simulink model "Three_phase_transformer_simulation"  (R2013b)
settings: Solver=ode45  StartTime=0.0  StopTime=0.1  RelTol=1e-3
libraries: powerlib x123
settings Model: Creator=Talha Israr  LastModifiedBy=Talha Israr

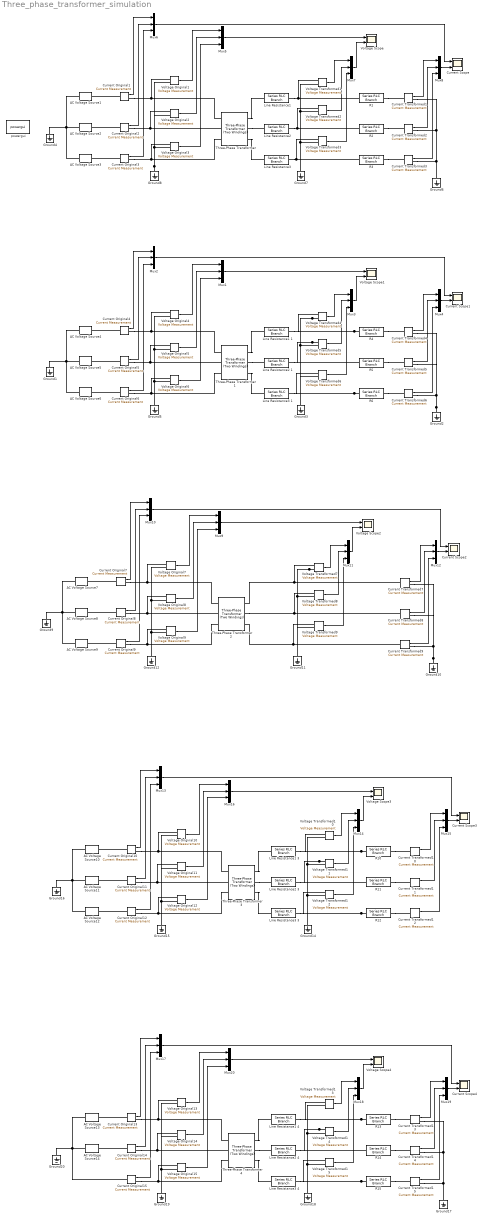
== system Three_phase_transformer_simulation ==
  AC Voltage Source{1,4,7,10,13} (5 alike) : powerlib/Electrical Sources/AC Voltage Source  Amplitude=220  Phase=0  Frequency=50  SampleTime=0  Measurements=None
  AC Voltage Source{2,5,8,11,14} (5 alike) : powerlib/Electrical Sources/AC Voltage Source  Amplitude=220  Phase=120  Frequency=50  SampleTime=0  Measurements=None
  AC Voltage Source{3,6,9,12} (4 alike) : powerlib/Electrical Sources/AC Voltage Source  Amplitude=220  Phase=240  Frequency=50  SampleTime=0  Measurements=None
  Current Original{1..15} (15 alike) : powerlib/Measurements/Current Measurement  PhasorSimulation=off  OutputType=Complex  PSBequivalent=0
  Current Scope{,1..4} (5 alike) : Scope  NumInputPorts=2
      Current Scope settings: YMin=-225~-1.25  YMax=300~1.5  MaxDataPoints=300000
      Current Scope1 settings: YMin=-225~-1.25  YMax=300~1.5  SaveName=ScopeData2  MaxDataPoints=300000
      Current Scope2 settings: YMin=-225~-1.25  YMax=300~1.5  SaveName=ScopeData4  MaxDataPoints=300000
      Current Scope3 settings: YMin=-225~-1.25  YMax=300~1.5  SaveName=ScopeData6  MaxDataPoints=300000
      Current Scope4 settings: YMin=-225~-1.25  YMax=300~1.5  SaveName=ScopeData8  MaxDataPoints=300000
  Current Transformed{1..15} (15 alike) : powerlib/Measurements/Current Measurement  PhasorSimulation=off  OutputType=Complex  PSBequivalent=0
  Ground{1..12,14..20} (19 alike) : powerlib/Elements/Ground  LConnTagsString=a
  Line Resistance1 {,1,3..4} (4 alike) : powerlib/Elements/Series RLC Branch  LConnTagsString=__new0  RConnTagsString=__new0  BranchType=R  Resistance=5  Inductance=1e-3  SetiL0=off  InitialCurrent=0  Capacitance=1e-6  Setx0=off  InitialVoltage=0  Measurements=None
  Line Resistance2 {,1,3..4} (4 alike) : powerlib/Elements/Series RLC Branch  LConnTagsString=__new0  RConnTagsString=__new0  BranchType=R  Resistance=5  Inductance=1e-3  SetiL0=off  InitialCurrent=0  Capacitance=1e-6  Setx0=off  InitialVoltage=0  Measurements=None
  Line Resistance3 {,1,3..4} (4 alike) : powerlib/Elements/Series RLC Branch  LConnTagsString=__new0  RConnTagsString=__new0  BranchType=R  Resistance=5  Inductance=2e-3  SetiL0=off  InitialCurrent=0  Capacitance=1e-6  Setx0=off  InitialVoltage=0  Measurements=None
  Mux{1..20} (20 alike) : Mux  Inputs=3
  R{1..2,10..11,13..14} (6 alike) : powerlib/Elements/Series RLC Branch  LConnTagsString=__new0  RConnTagsString=__new0  BranchType=R  Resistance=100  Inductance=1e-3  SetiL0=off  InitialCurrent=0  Capacitance=1e-6  Setx0=off  InitialVoltage=0  Measurements=None
  R12 : powerlib/Elements/Series RLC Branch  LConnTagsString=__new0  RConnTagsString=__new0  BranchType=R  Resistance=100  Inductance=2e-3  SetiL0=off  InitialCurrent=0  Capacitance=1e-6  Setx0=off  InitialVoltage=0  Measurements=None
  R15 : powerlib/Elements/Series RLC Branch  LConnTagsString=__new0  RConnTagsString=__new0  BranchType=R  Resistance=100  Inductance=2e-3  SetiL0=off  InitialCurrent=0  Capacitance=1e-6  Setx0=off  InitialVoltage=0  Measurements=None
  R3 : powerlib/Elements/Series RLC Branch  LConnTagsString=__new0  RConnTagsString=__new0  BranchType=R  Resistance=100  Inductance=2e-3  SetiL0=off  InitialCurrent=0  Capacitance=1e-6  Setx0=off  InitialVoltage=0  Measurements=None
  R4 : powerlib/Elements/Series RLC Branch  LConnTagsString=__new0  RConnTagsString=__new0  BranchType=RLC  Resistance=100  Inductance=5e-3  SetiL0=off  InitialCurrent=0  Capacitance=2e-6  Setx0=off  InitialVoltage=0  Measurements=None
  R5 : powerlib/Elements/Series RLC Branch  LConnTagsString=__new0  RConnTagsString=__new0  BranchType=RLC  Resistance=100  Inductance=5e-3  SetiL0=off  InitialCurrent=0  Capacitance=2e-6  Setx0=off  InitialVoltage=0  Measurements=None
  R6 : powerlib/Elements/Series RLC Branch  LConnTagsString=__new0  RConnTagsString=__new0  BranchType=RLC  Resistance=100  Inductance=5e-3  SetiL0=off  InitialCurrent=0  Capacitance=2e-6  Setx0=off  InitialVoltage=0  Measurements=None
  Three-Phase Transformer {,1..2,4} (4 alike) : powerlib/Elements/Three-Phase Transformer (Two Windings)  Winding1Connection=Y  UNITS=pu  NominalPower=[ 250e6 , 60 ]  Winding1=[ 220e3 , 0.002 , 0.08 ]  Winding2Connection=Y  Winding2=[ 12e3 , 0.002 , 0.08 ]  SetSaturation=off  Rm=500  Lm=500  Saturation=[ 0,0 ; 0.0024,1.2 ; 1.0,1.52 ]  Hysteresis=off  DataFile='hysteresis'  SetInitialFlux=off  InitialFluxes=[ 0.8 , -0.8 , 0.7 ]  Measurements=None  MoreParameters=off  BreakLoop=off  DataType=off  TransfoNumber=1
  Three-Phase Transformer 3 : powerlib/Elements/Three-Phase Transformer (Two Windings)  Winding1Connection=Yg  UNITS=pu  NominalPower=[ 250e6 , 60 ]  Winding1=[ 220e3 , 0.002 , 0.08 ]  Winding2Connection=Yg  Winding2=[ 12e3 , 0.002 , 0.08 ]  SetSaturation=off  Rm=500  Lm=500  Saturation=[ 0,0 ; 0.0024,1.2 ; 1.0,1.52 ]  Hysteresis=off  DataFile='hysteresis'  SetInitialFlux=off  InitialFluxes=[ 0.8 , -0.8 , 0.7 ]  Measurements=None  MoreParameters=off  BreakLoop=off  DataType=off  TransfoNumber=1
  Voltage Original{1..15} (15 alike) : powerlib/Measurements/Voltage Measurement  PhasorSimulation=off  OutputType=Complex  PSBequivalent=0
  Voltage Scope{,1..4} (5 alike) : Scope  NumInputPorts=2
      Voltage Scope settings: YMin=-225~-1.25  YMax=300~1.5  MaxDataPoints=300000
      Voltage Scope1 settings: YMin=-225~-1.25  YMax=300~1.5  SaveName=ScopeData3  MaxDataPoints=300000
      Voltage Scope2 settings: YMin=-225~-1.25  YMax=300~1.5  SaveName=ScopeData5  MaxDataPoints=300000
      Voltage Scope3 settings: YMin=-225~-1.25  YMax=300~1.5  SaveName=ScopeData7  MaxDataPoints=300000
      Voltage Scope4 settings: YMin=-225~-1.25  YMax=300~1.5  SaveName=ScopeData9  MaxDataPoints=300000
  Voltage Transformed{1..15} (15 alike) : powerlib/Measurements/Voltage Measurement  PhasorSimulation=off  OutputType=Complex  PSBequivalent=0
  powergui : powerlib/powergui  Priority=1  SimulationMode=Continuous  SolverType=Tustin  SampleTime=50e-6  frequency=60  SPID=off  DisableSnubberDevices=off  DisableRonSwitches=off  DisableVfSwitches=off  SwTol=0  Interpol=off  DisplayEquations=off  frequencyindice=50  Pbase=100e6  ErrMax=1e-4  Iterations=50  UnitsV=kV  UnitsW=MW  FunctionMessages=off  echomessages=off  HookPort=off  EnableUseOfTLC=off  x0status=blocks  RestoreLinks=warning  ResistiveCurrentMeasurement=off  Frange=[0:2:500]  Ylog=off  Xlog=on  ShowGrid=off  save=off  variable=ZData  ZoomFFT=off  StartTime=0.0  cycles=1  DisplayStyle=1  fundamental=60  FreqAxis=off  MaxFrequency=1000  frequencyindicesteady=1  RmsSteady=1  display=off  Ts=0  methode=off
  wires:
  Current Original1/1 -> Mux6/1
  Current Original2/1 -> Mux6/2
  Current Original3/1 -> Mux6/3
  Voltage Transformed1/1 -> Mux7/1
  Voltage Transformed2/1 -> Mux7/2
  Voltage Transformed3/1 -> Mux7/3
  Current Transformed3/1 -> Mux8/3
  Current Transformed2/1 -> Mux8/2
  Current Transformed1/1 -> Mux8/1
  Mux6/1 -> Current Scope/1
  Mux8/1 -> Current Scope/2
  Mux5/1 -> Voltage Scope/1
  Mux7/1 -> Voltage Scope/2
  Voltage Original3/1 -> Mux5/3
  Voltage Original2/1 -> Mux5/2
  Voltage Original1/1 -> Mux5/1
  Current Original4/1 -> Mux2/1
  Current Original5/1 -> Mux2/2
  Current Original6/1 -> Mux2/3
  Voltage Transformed4/1 -> Mux3/1
  Voltage Transformed5/1 -> Mux3/2
  Voltage Transformed6/1 -> Mux3/3
  Current Transformed6/1 -> Mux4/3
  Current Transformed5/1 -> Mux4/2
  Current Transformed4/1 -> Mux4/1
  Mux2/1 -> Current Scope1/1
  Mux4/1 -> Current Scope1/2
  Mux1/1 -> Voltage Scope1/1
  Mux3/1 -> Voltage Scope1/2
  Voltage Original6/1 -> Mux1/3
  Voltage Original5/1 -> Mux1/2
  Voltage Original4/1 -> Mux1/1
  Current Original7/1 -> Mux10/1
  Current Original8/1 -> Mux10/2
  Current Original9/1 -> Mux10/3
  Voltage Transformed7/1 -> Mux11/1
  Voltage Transformed8/1 -> Mux11/2
  Voltage Transformed9/1 -> Mux11/3
  Current Transformed9/1 -> Mux12/3
  Current Transformed8/1 -> Mux12/2
  Current Transformed7/1 -> Mux12/1
  Mux10/1 -> Current Scope2/1
  Mux12/1 -> Current Scope2/2
  Mux9/1 -> Voltage Scope2/1
  Mux11/1 -> Voltage Scope2/2
  Voltage Original9/1 -> Mux9/3
  Voltage Original8/1 -> Mux9/2
  Voltage Original7/1 -> Mux9/1
  Current Original10/1 -> Mux13/1
  Current Original11/1 -> Mux13/2
  Current Original12/1 -> Mux13/3
  Voltage Transformed10/1 -> Mux14/1
  Voltage Transformed11/1 -> Mux14/2
  Voltage Transformed12/1 -> Mux14/3
  Current Transformed12/1 -> Mux15/3
  Current Transformed11/1 -> Mux15/2
  Current Transformed10/1 -> Mux15/1
  Mux13/1 -> Current Scope3/1
  Mux15/1 -> Current Scope3/2
  Mux16/1 -> Voltage Scope3/1
  Mux14/1 -> Voltage Scope3/2
  Voltage Original12/1 -> Mux16/3
  Voltage Original11/1 -> Mux16/2
  Voltage Original10/1 -> Mux16/1
  Current Original13/1 -> Mux17/1
  Current Original14/1 -> Mux17/2
  Current Original15/1 -> Mux17/3
  Voltage Transformed13/1 -> Mux18/1
  Voltage Transformed14/1 -> Mux18/2
  Voltage Transformed15/1 -> Mux18/3
  Current Transformed15/1 -> Mux19/3
  Current Transformed14/1 -> Mux19/2
  Current Transformed13/1 -> Mux19/1
  Mux17/1 -> Current Scope4/1
  Mux19/1 -> Current Scope4/2
  Mux20/1 -> Voltage Scope4/1
  Mux18/1 -> Voltage Scope4/2
  Voltage Original15/1 -> Mux20/3
  Voltage Original14/1 -> Mux20/2
  Voltage Original13/1 -> Mux20/1
  connections:
  R2/LConn1 -- "Line Resistance2 "/RConn1 -- Voltage Transformed2/LConn1
  AC Voltage Source2/LConn1 -- Ground4/LConn1 -- AC Voltage Source3/LConn1 -- AC Voltage Source1/LConn1
  Current Transformed1/RConn1 -- Current Transformed2/RConn1 -- Current Transformed3/RConn1 -- Ground6/LConn1
  Voltage Transformed3/LConn2 -- Ground7/LConn1 -- Voltage Transformed2/LConn2 -- Voltage Transformed1/LConn2
  Voltage Original2/LConn1 -- "Three-Phase Transformer "/LConn2 -- Current Original2/RConn1
  "Three-Phase Transformer "/LConn3 -- Voltage Original3/LConn1 -- Current Original3/RConn1
  Voltage Original1/LConn1 -- "Three-Phase Transformer "/LConn1 -- Current Original1/RConn1
  Voltage Transformed1/LConn1 -- "Line Resistance1 "/RConn1 -- R1/LConn1
  Ground8/LConn1 -- Voltage Original3/LConn2 -- Voltage Original1/LConn2 -- Voltage Original2/LConn2
  Current Original1/LConn1 -- AC Voltage Source1/RConn1
  R3/RConn1 -- Current Transformed3/LConn1
  R2/RConn1 -- Current Transformed2/LConn1
  Current Original2/LConn1 -- AC Voltage Source2/RConn1
  Voltage Transformed3/LConn1 -- "Line Resistance3 "/RConn1 -- R3/LConn1
  Current Original3/LConn1 -- AC Voltage Source3/RConn1
  R1/RConn1 -- Current Transformed1/LConn1
  "Three-Phase Transformer "/RConn2 -- "Line Resistance2 "/LConn1
  "Three-Phase Transformer "/RConn3 -- "Line Resistance3 "/LConn1
  "Three-Phase Transformer "/RConn1 -- "Line Resistance1 "/LConn1
  Voltage Transformed5/LConn1 -- R5/LConn1 -- Line Resistance2 1/RConn1
  AC Voltage Source4/LConn1 -- AC Voltage Source5/LConn1 -- Ground1/LConn1 -- AC Voltage Source6/LConn1
  Ground2/LConn1 -- Current Transformed6/RConn1 -- Current Transformed4/RConn1 -- Current Transformed5/RConn1
  Voltage Transformed4/LConn2 -- Voltage Transformed5/LConn2 -- Voltage Transformed6/LConn2 -- Ground3/LConn1
  Current Original5/RConn1 -- Voltage Original5/LConn1 -- Three-Phase Transformer 1/LConn2
  Current Original6/RConn1 -- Three-Phase Transformer 1/LConn3 -- Voltage Original6/LConn1
  Current Original4/RConn1 -- Voltage Original4/LConn1 -- Three-Phase Transformer 1/LConn1
  R4/LConn1 -- Voltage Transformed4/LConn1 -- Line Resistance1 1/RConn1
  Voltage Original5/LConn2 -- Voltage Original4/LConn2 -- Ground5/LConn1 -- Voltage Original6/LConn2
  R6/LConn1 -- Voltage Transformed6/LConn1 -- Line Resistance3 1/RConn1
  Current Original5/LConn1 -- AC Voltage Source5/RConn1
  R6/RConn1 -- Current Transformed6/LConn1
  R4/RConn1 -- Current Transformed4/LConn1
  R5/RConn1 -- Current Transformed5/LConn1
  Current Original4/LConn1 -- AC Voltage Source4/RConn1
  Current Original6/LConn1 -- AC Voltage Source6/RConn1
  Three-Phase Transformer 1/RConn2 -- Line Resistance2 1/LConn1
  Three-Phase Transformer 1/RConn3 -- Line Resistance3 1/LConn1
  Three-Phase Transformer 1/RConn1 -- Line Resistance1 1/LConn1
  AC Voltage Source7/LConn1 -- AC Voltage Source8/LConn1 -- Ground9/LConn1 -- AC Voltage Source9/LConn1
  Ground10/LConn1 -- Current Transformed9/RConn1 -- Current Transformed7/RConn1 -- Current Transformed8/RConn1
  Voltage Transformed7/LConn2 -- Voltage Transformed8/LConn2 -- Voltage Transformed9/LConn2 -- Ground11/LConn1
  Current Original8/RConn1 -- Voltage Original8/LConn1 -- Three-Phase Transformer 2/LConn2
  Current Original9/RConn1 -- Three-Phase Transformer 2/LConn3 -- Voltage Original9/LConn1
  Current Original7/RConn1 -- Voltage Original7/LConn1 -- Three-Phase Transformer 2/LConn1
  Voltage Original8/LConn2 -- Voltage Original7/LConn2 -- Ground12/LConn1 -- Voltage Original9/LConn2
  Current Original8/LConn1 -- AC Voltage Source8/RConn1
  Current Original7/LConn1 -- AC Voltage Source7/RConn1
  Current Original9/LConn1 -- AC Voltage Source9/RConn1
  Current Transformed8/LConn1 -- Three-Phase Transformer 2/RConn2 -- Voltage Transformed8/LConn1
  Voltage Transformed9/LConn1 -- Current Transformed9/LConn1 -- Three-Phase Transformer 2/RConn3
  Voltage Transformed7/LConn1 -- Three-Phase Transformer 2/RConn1 -- Current Transformed7/LConn1
  Voltage Transformed11/LConn1 -- R11/LConn1 -- Line Resistance2 3/RConn1
  AC Voltage Source10/LConn1 -- AC Voltage Source11/LConn1 -- Ground16/LConn1 -- AC Voltage Source12/LConn1
  Ground14/LConn1 -- Voltage Transformed12/LConn2 -- Voltage Transformed11/LConn2 -- Voltage Transformed10/LConn2
  Current Original11/RConn1 -- Voltage Original11/LConn1 -- Three-Phase Transformer 3/LConn2
  Current Original12/RConn1 -- Three-Phase Transformer 3/LConn3 -- Voltage Original12/LConn1
  Current Original10/RConn1 -- Voltage Original10/LConn1 -- Three-Phase Transformer 3/LConn1
  R10/LConn1 -- Voltage Transformed10/LConn1 -- Line Resistance1 3/RConn1
  Voltage Original12/LConn2 -- Ground15/LConn1 -- Voltage Original10/LConn2 -- Voltage Original11/LConn2
  R12/LConn1 -- Voltage Transformed12/LConn1 -- Line Resistance3 3/RConn1
  Current Original10/LConn1 -- AC Voltage Source10/RConn1
  Three-Phase Transformer 3/RConn3 -- Line Resistance3 3/LConn1
  R10/RConn1 -- Current Transformed10/LConn1
  Current Original12/LConn1 -- AC Voltage Source12/RConn1
  R12/RConn1 -- Current Transformed12/LConn1
  Three-Phase Transformer 3/RConn1 -- Line Resistance1 3/LConn1
  R11/RConn1 -- Current Transformed11/LConn1
  Current Original11/LConn1 -- AC Voltage Source11/RConn1
  Three-Phase Transformer 3/RConn2 -- Line Resistance2 3/LConn1
  Voltage Transformed14/LConn1 -- R14/LConn1 -- Line Resistance2 4/RConn1
  Current Transformed14/RConn1 -- Current Transformed13/RConn1 -- Current Transformed15/RConn1 -- Ground17/LConn1
  Ground18/LConn1 -- Voltage Transformed15/LConn2 -- Voltage Transformed14/LConn2 -- Voltage Transformed13/LConn2
  Current Original14/RConn1 -- Voltage Original14/LConn1 -- Three-Phase Transformer 4/LConn2
  Current Original15/RConn1 -- Three-Phase Transformer 4/LConn3 -- Voltage Original15/LConn1
  Current Original13/RConn1 -- Voltage Original13/LConn1 -- Three-Phase Transformer 4/LConn1
  R13/LConn1 -- Voltage Transformed13/LConn1 -- Line Resistance1 4/RConn1
  Voltage Original15/LConn2 -- Ground19/LConn1 -- Voltage Original13/LConn2 -- Voltage Original14/LConn2
  R15/LConn1 -- Voltage Transformed15/LConn1 -- Line Resistance3 4/RConn1
  Current Original13/LConn1 -- AC Voltage Source13/RConn1
  Three-Phase Transformer 4/RConn3 -- Line Resistance3 4/LConn1
  R13/RConn1 -- Current Transformed13/LConn1
  AC Voltage Source13/LConn1 -- Current Original15/LConn1 -- AC Voltage Source14/LConn1 -- Ground20/LConn1
  R15/RConn1 -- Current Transformed15/LConn1
  Three-Phase Transformer 4/RConn1 -- Line Resistance1 4/LConn1
  R14/RConn1 -- Current Transformed14/LConn1
  Current Original14/LConn1 -- AC Voltage Source14/RConn1
  Three-Phase Transformer 4/RConn2 -- Line Resistance2 4/LConn1
